simulink model "pv_mod_noct"  (R2025a)
settings: Solver=ode8  StartTime=0.0  StopTime=5  FixedStep=1e-4  MaxStep=0.2  RelTol=1e-3
libraries: SignalEditorBlockLib x1, simulink x1
settings Model: Creator=vrsam  LastModifiedBy=imaka
settings DebuggingCC: AlgebraicLoopMsg=none

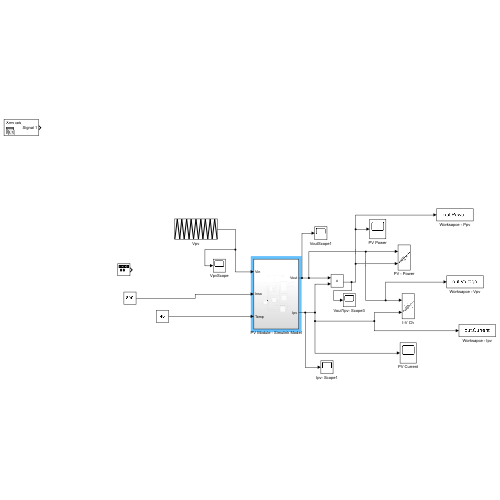
[thumbnail: Simulink's stored preview of the top-level diagram]
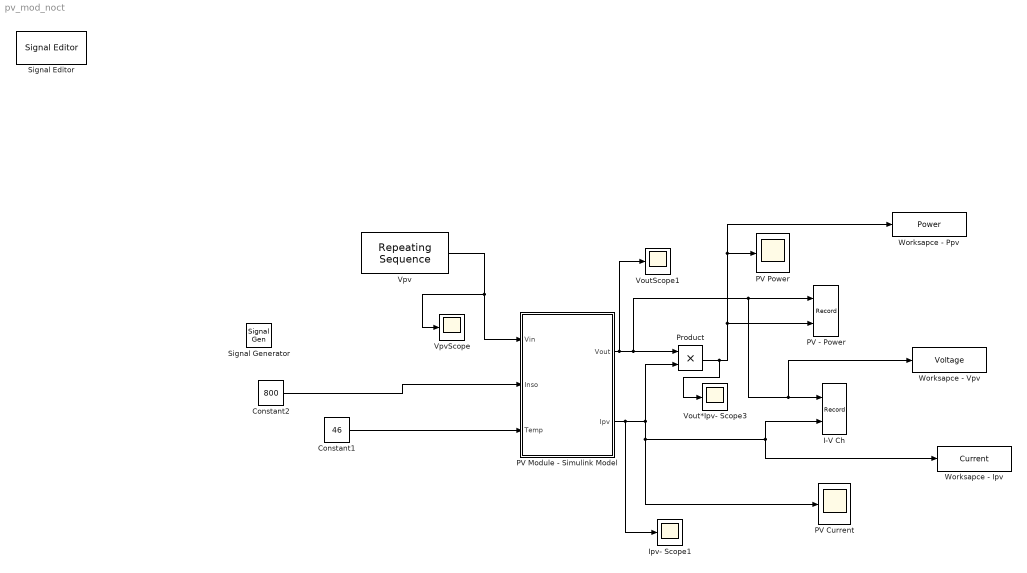
== system pv_mod_noct ==
  Constant1 : Constant  Value=46
  Constant2 : Constant  Value=800
  I-V Ch : Record  NumPorts=2.0  FileSettingsInternal="{\"entries\":[{\"content\":{\"excelSettings\":{\"content\":{},\"type\":\"Streamout.ExcelSettings\"},\"parquetSettings\":{\"content\":{},\"type\":\"Streamout.ParquetSettings\"}},\"type\":\"Streamout.FileSettingStorage\",\"uuid\":\"\"}],\"packageUris\":[\"http:\\/\\/schema.mathworks.com\\/mf0\\/streamout_blocks\\/R2020a\"],\"version\":\"1.0\"}"  FrameSettings=[0, 0]  Layout=[1 1]  SignalsInternal="{\"entries\":[{\"content\":{\"signals\":[{\"content\":{\"blockPath\":[],\"dimensions\":[1],\"domain\":\"\",\"lineColor\":\"#edb120\",\"lineWidth\":2,\"plots\":[ 1 ],\"port\":1,\"sid\":[\"\"],\"signalID\":1,\"signalName\":\"PV Module - Simulink Model:1\"},\"type\":\"RecordBlkView.Signal\",\"uuid\":\"\"},{\"content\":{\"blockPath\":[],\"dimensions\":[1],\"domain\":\"\",\"lineColor\":\"#7e2f8e\",\"lineWidth\":2,\"plots\":[ 1 ],\"port\":2,\"sid\":[\"\"],\"signalID\":2,\"signalName\":\"PV Module - Simulink Model:2\"},\"type\":\"RecordBlkView.Signal\",\"uuid\":\"\"}]},\"type\":\"RecordBlkView.InputSignals\",\"uuid\":\"\"}],\"packageUris\":[\"http:\\/\\/schema.mathworks.com\\/mf0\\/streamout_blocks\\/R2020a\"],\"version\":\"1.0\"}"  VisualizationBindings="{\"xyplotplugin\":{\"info\":[{\"series\":[{\"bindingParametersList\":[{\"parameter\":\"X-Axis\",\"signalID\":1,\"signalName\":\"PV Module - Simulink Model:1\"},{\"parameter\":\"Y-Axis\",\"signalID\":2,\"signalName\":\"PV Module - Simulink Model:2\"}],\"seriesID\":0}],\"subplotID\":1}]}}"  CompatibilityTag=XY
  Ipv- Scope1 : Scope
      settings: ActiveDisplayYMinimum=-121.22534417187291  ActiveDisplayYMaximum=71.2231278952772  DataLoggingVariableName=ScopeData5
  PV - Power : Record  NumPorts=2.0  FileSettingsInternal="{\"entries\":[{\"content\":{\"excelSettings\":{\"content\":{},\"type\":\"Streamout.ExcelSettings\"},\"parquetSettings\":{\"content\":{},\"type\":\"Streamout.ParquetSettings\"}},\"type\":\"Streamout.FileSettingStorage\",\"uuid\":\"\"}],\"packageUris\":[\"http:\\/\\/schema.mathworks.com\\/mf0\\/streamout_blocks\\/R2020a\"],\"version\":\"1.0\"}"  FrameSettings=[0, 0]  Layout=[1 1]  SignalsInternal="{\"entries\":[{\"content\":{\"signals\":[{\"content\":{\"blockPath\":[],\"dimensions\":[1],\"domain\":\"\",\"lineColor\":\"#77ac30\",\"lineWidth\":2,\"plots\":[ 1 ],\"port\":1,\"sid\":[\"\"],\"signalID\":1,\"signalName\":\"PV Module - Simulink Model:1\"},\"type\":\"RecordBlkView.Signal\",\"uuid\":\"\"},{\"content\":{\"blockPath\":[],\"dimensions\":[1],\"domain\":\"\",\"lineColor\":\"#4dbeee\",\"lineWidth\":2,\"plots\":[ 1 ],\"port\":2,\"sid\":[\"\"],\"signalID\":2,\"signalName\":\"Product\"},\"type\":\"RecordBlkView.Signal\",\"uuid\":\"\"}]},\"type\":\"RecordBlkView.InputSignals\",\"uuid\":\"\"}],\"packageUris\":[\"http:\\/\\/schema.mathworks.com\\/mf0\\/streamout_blocks\\/R2020a\"],\"version\":\"1.0\"}"  VisualizationBindings="{\"xyplotplugin\":{\"info\":[{\"series\":[{\"bindingParametersList\":[{\"parameter\":\"X-Axis\",\"signalID\":1,\"signalName\":\"PV Module - Simulink Model:1\"},{\"parameter\":\"Y-Axis\",\"signalID\":2,\"signalName\":\"Product\"}],\"seriesID\":0}],\"subplotID\":1}]}}"  CompatibilityTag=XY
  PV Current : Scope
      settings: ActiveDisplayYMinimum=-1  ActiveDisplayYMaximum=1
  PV Module - Simulink Model : Subsystem
  PV Power : Scope
      settings: ActiveDisplayYMinimum=-1  ActiveDisplayYMaximum=1
  Product : Product
  Signal Generator : SignalGenerator  Units=rad/sec
  Signal Editor : SignalEditorBlockLib/Signal Editor  FileName=sig_ed1.mat  ActiveScenario=Scenario  ActiveSignal=Signal 1  IsBus=off  OutputBusObjectStr=Bus: BusObject  SampleTime=0  ZeroCross=off  OutputAfterFinalValue=Setting to zero  Unit=inherit  PreserveSignalName=on  ApplySigPropsToAllScenarios=on  ApplySigPropsToAllSignals=off  SignalPropertySource=Dialog parameters
  Vout*Ipv- Scope3 : Scope
      settings: ActiveDisplayYMinimum=-125.61185821134148  ActiveDisplayYMaximum=77.626100345613452  DataLoggingVariableName=ScopeData4
  VoutScope1 : Scope
      settings: ActiveDisplayYMinimum=-27.403901477051193  ActiveDisplayYMaximum=27.478899349575812  DataLoggingVariableName=ScopeData3
  Vpv : simulink/Sources/Repeating Sequence  rep_seq_t=[0 1 2 3 4 5 6]  rep_seq_y=[0 19.5 0 19.5 0 19.5 0]
  VpvScope : Scope
      settings: ActiveDisplayYMinimum=-27.403901477051193  ActiveDisplayYMaximum=27.478899349575812  DataLoggingVariableName=ScopeData2
  Worksapce - Ipv : ToWorkspace  VariableName=Current  SaveFormat=Timeseries  SampleTime=-1
  Worksapce - Ppv : ToWorkspace  VariableName=Power  SaveFormat=Timeseries  SampleTime=-1
  Worksapce - Vpv : ToWorkspace  VariableName=Voltage  SaveFormat=Timeseries  SampleTime=-1
  wires:
  PV Module - Simulink Model/2(Ipv) -> Ipv- Scope1/1, I-V Ch/2, Worksapce - Ipv/1, PV Current/1, Product/2
  PV Module - Simulink Model/1(Vout) -> VoutScope1/1, Worksapce - Vpv/1, I-V Ch/1, PV - Power/1, Product/1
  Product/1 -> Vout*Ipv- Scope3/1, Worksapce - Ppv/1, PV Power/1, PV - Power/2
  Vpv/1 -> PV Module - Simulink Model/1(Vin), VpvScope/1
  Constant1/1 -> PV Module - Simulink Model/3(Temp)
  Constant2/1 -> PV Module - Simulink Model/2(Inso)

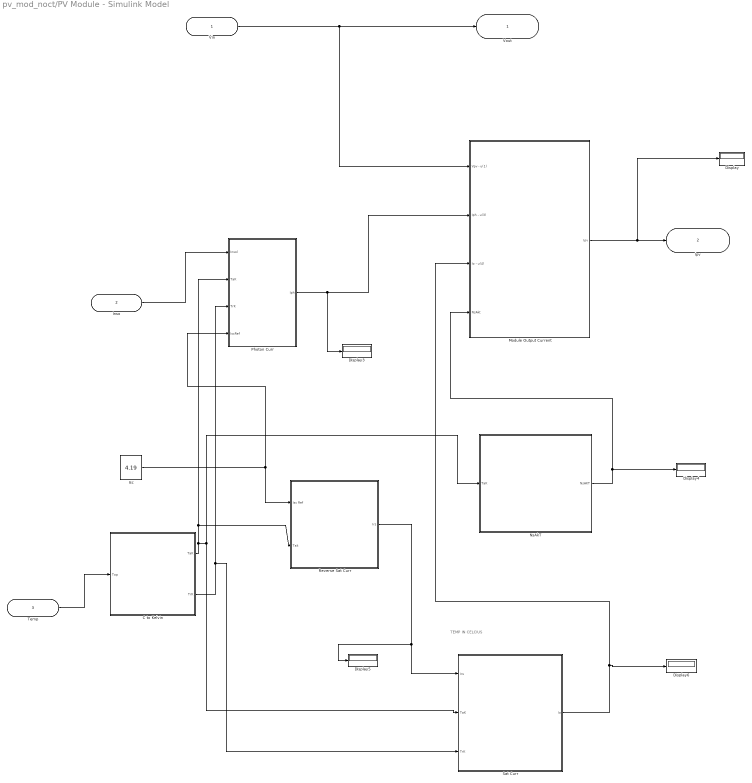
== system pv_mod_noct/PV Module - Simulink Model ==
  note: TEMP IN CELCIUS
  Vin : Inport
  Inso : Inport  Port=2
  Temp : Inport  Port=3
  C to Kelvin : Subsystem
  Display{,3..6} (5 alike) : Display
  Isc : Constant  Value=4.19
  Module Output Current : Subsystem
  NsAkT : Subsystem
  Photon Curr : Subsystem
  Reverse Sat Curr : Subsystem
  Sat Curr : Subsystem
  Vout : Outport
  Ipv : Outport  Port=2
  wires:
  NsAkT/1(NsAKT) -> Display4/1, Module Output Current/4(NsAkt)
  Inso/1 -> Photon Curr/1(Insol)
  Vin/1 -> Module Output Current/1(Vpv - u(1)), Vout/1
  Module Output Current/1(Ipv) -> Display/1, Ipv/1
  Sat Curr/1(Io) -> Display6/1, Module Output Current/3(Io - u(4))
  Photon Curr/1(Iph) -> Display3/1, Module Output Current/2(Iph - u(3))
  Temp/1 -> C to Kelvin/1(Top)
  C to Kelvin/1(TaK) -> Photon Curr/2(TaK), Reverse Sat Curr/2(Tak), Sat Curr/2(TaK), NsAkT/1(TaK)
  Reverse Sat Curr/1(Irs) -> Display5/1, Sat Curr/1(Irs)
  Isc/1 -> Reverse Sat Curr/1(Isc Ref), Photon Curr/4(IscRef)
  C to Kelvin/2(TrK) -> Photon Curr/3(TrK), Sat Curr/3(TrK)

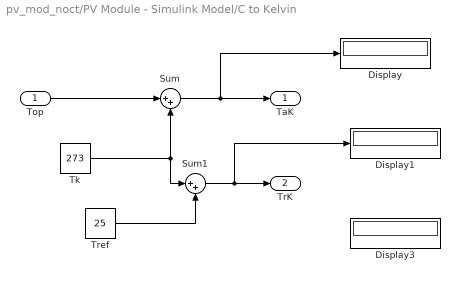
== system pv_mod_noct/PV Module - Simulink Model/C to Kelvin ==
  Top : Inport
  Display : Display
  Display1 : Display
  Display3 : Display
  Sum : Sum  Inputs=|++
  Sum1 : Sum  Inputs=|++
  Tk : Constant  Value=273
  Tref : Constant  Value=25
  TaK : Outport
  TrK : Outport  Port=2
  wires:
  Top/1 -> Sum/1
  Sum/1 -> Display/1, TaK/1
  Tk/1 -> Sum1/1, Sum/2
  Tref/1 -> Sum1/2
  Sum1/1 -> TrK/1, Display1/1

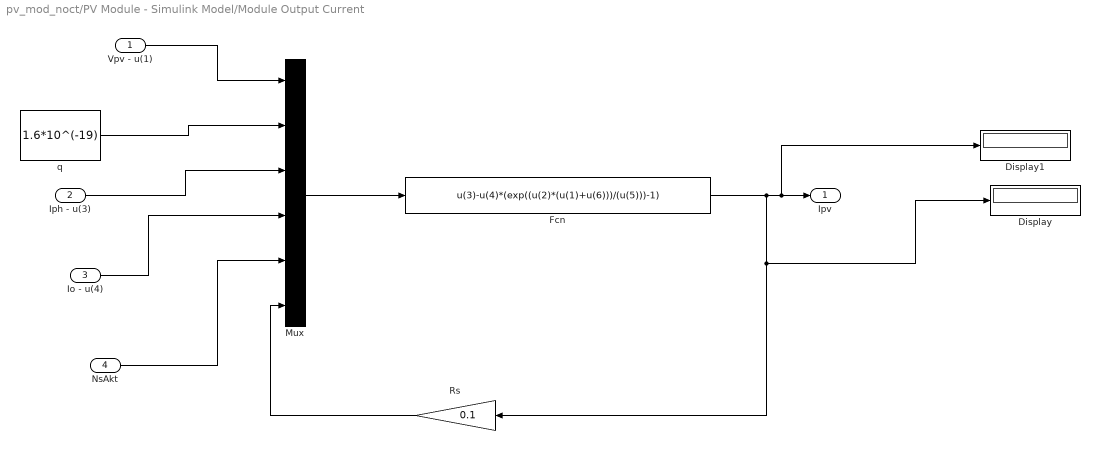
== system pv_mod_noct/PV Module - Simulink Model/Module Output Current ==
  Vpv - u(1) : Inport
  Iph - u(3) : Inport  Port=2
  Io - u(4) : Inport  Port=3
  NsAkt : Inport  Port=4
  Display : Display
  Display1 : Display
  Fcn : Fcn  Expr=u(3)-u(4)*(exp((u(2)*(u(1)+u(6)))/(u(5)))-1)
  Mux : Mux  Inputs=6
  Rs : Gain  Gain=0.1
  q : Constant  Value=1.6*10^(-19)
  Ipv : Outport
  wires:
  Vpv - u(1)/1 -> Mux/1
  q/1 -> Mux/2
  Iph - u(3)/1 -> Mux/3
  Io - u(4)/1 -> Mux/4
  NsAkt/1 -> Mux/5
  Mux/1 -> Fcn/1
  Fcn/1 -> Rs/1, Display/1, Display1/1, Ipv/1
  Rs/1 -> Mux/6

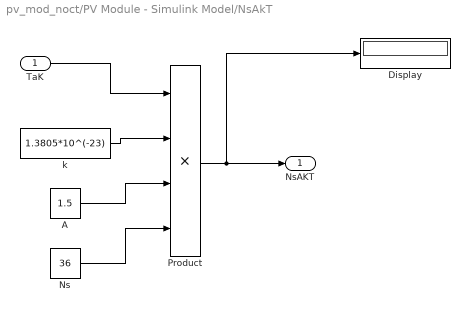
== system pv_mod_noct/PV Module - Simulink Model/NsAkT ==
  TaK : Inport
  A : Constant  Value=1.5
  Display : Display
  Ns : Constant  Value=36
  Product : Product  Inputs=4
  k : Constant  Value=1.3805*10^(-23)
  NsAKT : Outport
  wires:
  TaK/1 -> Product/1
  k/1 -> Product/2
  A/1 -> Product/3
  Ns/1 -> Product/4
  Product/1 -> Display/1, NsAKT/1

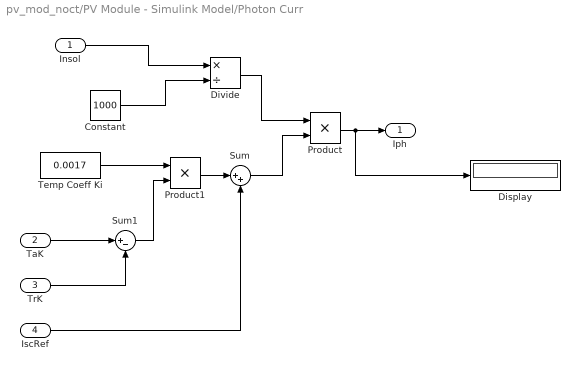
== system pv_mod_noct/PV Module - Simulink Model/Photon Curr ==
  Insol : Inport
  TaK : Inport  Port=2
  TrK : Inport  Port=3
  IscRef : Inport  Port=4
  Constant : Constant  Value=1000
  Display : Display
  Divide : Product  Inputs=*/
  Product : Product
  Product1 : Product
  Sum : Sum  Inputs=|++
  Sum1 : Sum  Inputs=|+-
  Temp Coeff Ki : Constant  Value=0.0017
  Iph : Outport
  wires:
  Sum/1 -> Product/2
  Product/1 -> Display/1, Iph/1
  Product1/1 -> Sum/1
  Temp Coeff Ki/1 -> Product1/1
  Sum1/1 -> Product1/2
  TaK/1 -> Sum1/1
  TrK/1 -> Sum1/2
  IscRef/1 -> Sum/2
  Insol/1 -> Divide/1
  Constant/1 -> Divide/2
  Divide/1 -> Product/1

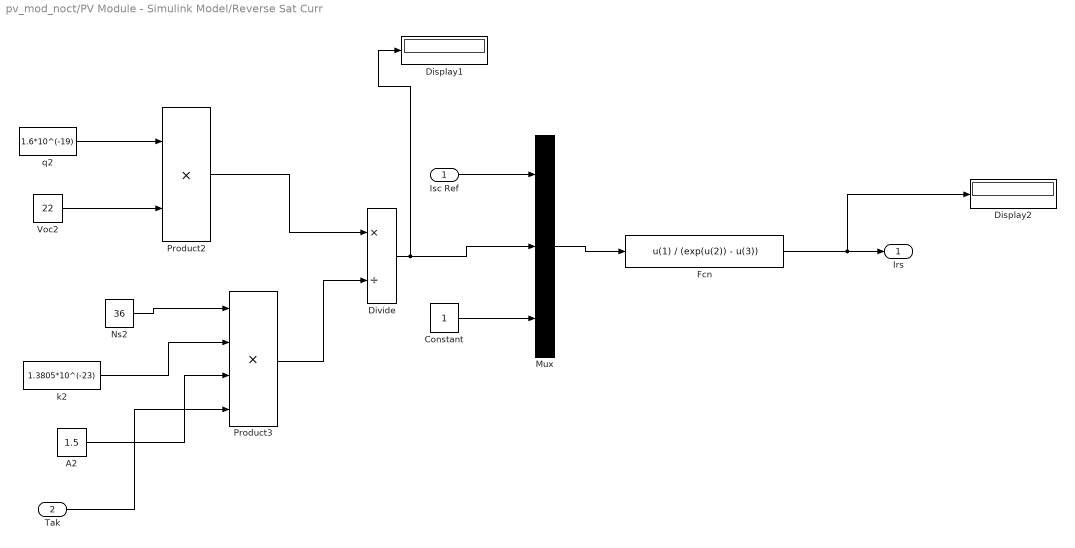
== system pv_mod_noct/PV Module - Simulink Model/Reverse Sat Curr ==
  Isc Ref : Inport
  Tak : Inport  Port=2
  A2 : Constant  Value=1.5
  Constant : Constant
  Display1 : Display
  Display2 : Display
  Divide : Product  Inputs=*/
  Fcn : Fcn  Expr=u(1) / (exp(u(2)) - u(3))
  Mux : Mux  Inputs=3
  Ns2 : Constant  Value=36
  Product2 : Product
  Product3 : Product  Inputs=4
  Voc2 : Constant  Value=22
  k2 : Constant  Value=1.3805*10^(-23)
  q2 : Constant  Value=1.6*10^(-19)
  Irs : Outport
  wires:
  Fcn/1 -> Display2/1, Irs/1
  Isc Ref/1 -> Mux/1
  Constant/1 -> Mux/3
  Mux/1 -> Fcn/1
  k2/1 -> Product3/2
  A2/1 -> Product3/3
  Tak/1 -> Product3/4
  Ns2/1 -> Product3/1
  q2/1 -> Product2/1
  Product2/1 -> Divide/1
  Divide/1 -> Mux/2, Display1/1
  Voc2/1 -> Product2/2
  Product3/1 -> Divide/2

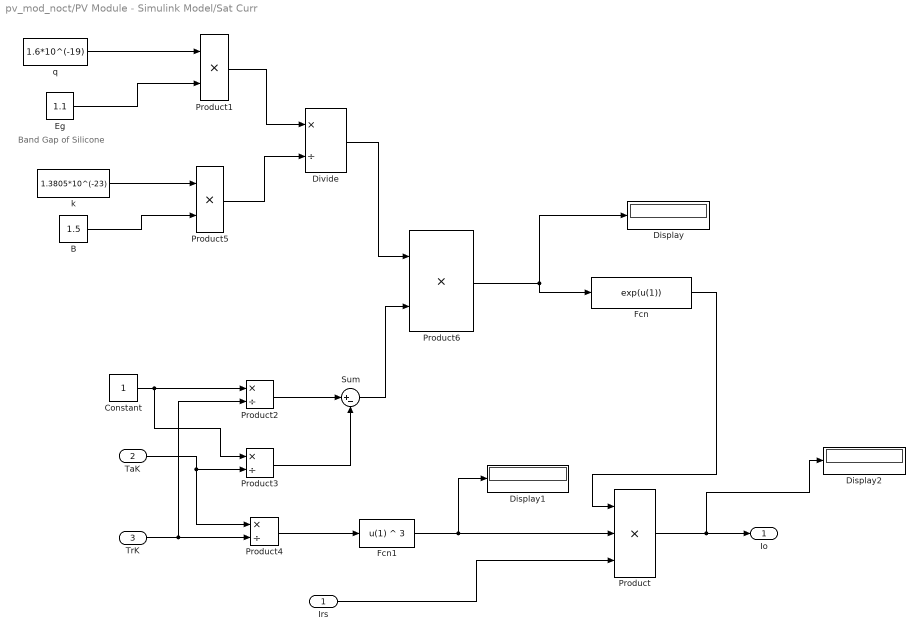
== system pv_mod_noct/PV Module - Simulink Model/Sat Curr ==
  note: Band Gap of Silicone
  Irs : Inport
  TaK : Inport  Port=2
  TrK : Inport  Port=3
  B : Constant  Value=1.5
  Constant : Constant
  Display : Display
  Display1 : Display
  Display2 : Display
  Divide : Product  Inputs=*/
  Eg : Constant  Value=1.1
  Fcn : Fcn  Expr=exp(u(1))
  Fcn1 : Fcn  Expr=u(1) ^ 3
  Product : Product  Inputs=3
  Product1 : Product
  Product2 : Product  Inputs=*/
  Product3 : Product  Inputs=*/
  Product4 : Product  Inputs=*/
  Product5 : Product
  Product6 : Product
  Sum : Sum  Inputs=|+-
  k : Constant  Value=1.3805*10^(-23)
  q : Constant  Value=1.6*10^(-19)
  Io : Outport
  wires:
  Product/1 -> Display2/1, Io/1
  Fcn/1 -> Product/1
  Product6/1 -> Fcn/1, Display/1
  Irs/1 -> Product/3
  Product2/1 -> Sum/1
  Product3/1 -> Sum/2
  Constant/1 -> Product3/1, Product2/1
  TaK/1 -> Product4/1, Product3/2
  TrK/1 -> Product2/2, Product4/2
  Product4/1 -> Fcn1/1
  Fcn1/1 -> Display1/1, Product/2
  q/1 -> Product1/1
  Eg/1 -> Product1/2
  k/1 -> Product5/1
  B/1 -> Product5/2
  Product1/1 -> Divide/1
  Product5/1 -> Divide/2
  Divide/1 -> Product6/1
  Sum/1 -> Product6/2
